simulink model "ChimeIndicatorOutput"  (R2018b)
settings: Solver=FixedStepDiscrete  StartTime=0.0  StopTime=10.0  FixedStep=0.01  RelTol=1e-3
undefined symbols (not defined in the file or in its folder): f, h, IfVeSMSeStNumConfig, KeSMSbMdChime1Enable_Val, KeSMSbSRSPosNumConfig_Val, KeSMSuChmReqDurmTm_Val, KeSMSuChmReqIntlTm_Val, KeSMSwModeChimeReqTm_Val, KeSMSwSRSActiveValidTm_Val, SRSIndicatorStat1
libraries: MSMLib x27
(part 2 of 2)

== stateflow chart ChimeIndicatorOutput/ChimeIndicatorOutputRunnable_sys/Subsystem/SRSIndicator/Chart ==
  state PowerOn
  state Slct_None
    en:
    oSRSIndicatorStat = SRSIndicatorStat1.SRSIndicatorStat1_NoIndicator;
    oSRSMdSlctSwStat =0;
    oSRSMdSlctSwIndTyp = 0;
  state Slct_Avail
    state NotConfirm
      state ON
        en:
        oSRSIndicatorStat = iSlctSwStat;
        oSRSMdSlctSwStat = iSRSMdSlctSwReq_67_2;
        oSRSMdSlctSwIndTyp = 3;
      state OFF
        en:
        oSRSIndicatorStat = SRSIndicatorStat1.SRSIndicatorStat1_NoIndicator;
        oSRSMdSlctSwStat = 0;
        oSRSMdSlctSwIndTyp = 0;
      Slct_Avail.NotConfirm.ON -> Slct_Avail.NotConfirm.ON [order 2] : [hasChanged(iSlctSwStat) && (iSlctSwStat != SRSIndicatorStat1.SRSIndicatorStat1_NoIndicator)]
      Slct_Avail.NotConfirm.ON -> Slct_Avail.NotConfirm.OFF [order 3] : [after(iValideTm,tick)]
      (default) -> Slct_Avail.NotConfirm.ON
      Slct_Avail.NotConfirm.OFF -> Slct_Avail.NotConfirm.ON : [hasChanged(iSlctSwStat)]
    state Confirm
      en:
      oSRSMdSlctSwIndTyp = 1;
      du:
      oSRSIndicatorStat =ConfirmSRSIndicatorStat();
      state ON
        en:
        SRSMdSlctSwReq_67_2_temp = iSRSMdSlctSwReq_67_2;
      state OFF
        en:
        SRSMdSlctSwReq_67_2_temp = 0;
      Slct_Avail.Confirm.ON -> Slct_Avail.Confirm.ON [order 2] : [(iSRSMdSlctSwReq_67_2 != SRSMdSlctSwReq_67_2_temp) && (iSRSMdSlctSwReq_67_2 != 0)]
      (default) -> Slct_Avail.Confirm.OFF
      Slct_Avail.Confirm.OFF -> Slct_Avail.Confirm.ON : [iSRSMdSlctSwReq_67_2 != 0]
      Slct_Avail.Confirm.ON -> Slct_Avail.Confirm.OFF [order 1] : [after(iValideTm,tick)]
    (default) -> NotConfirm
    Confirm -> Slct_Avail.NotConfirm.OFF [order 2] : [(icurMode == MdTp1.MdTp_None)&&after(5,tick)]
    Slct_Avail.NotConfirm.ON -> Confirm [order 1] : [hasChangedTo(iIsActive,true)]
  note: // fail to start Mode for Avl invalid
  state out =ConfirmSRSIndicatorStat [function]
    (default) -> (junction 263)
    (junction 263) -> (junction 264) [order 1] : [iSRSMode == SRSCurMode1.SRSMode_EZEEntry]
    (junction 264) -> (junction 287) : {out = SRSIndicatorStat1.SRSIndicatorStat1_EzeEntry;}
    (junction 263) -> (junction 265) [order 2]
    (junction 265) -> (junction 266) [order 1] : [iSRSMode == SRSCurMode1.SRSMode_EzeExt]
    (junction 266) -> (junction 286) : {out = SRSIndicatorStat1.SRSIndicatorStat1_EzeExit;}
    (junction 265) -> (junction 267) [order 2]
    (junction 267) -> (junction 268) [order 1] : [iSRSMode == SRSCurMode1.SRSMode_LfVip]
    (junction 268) -> (junction 285) : {out = SRSIndicatorStat1.SRSIndicatorStat1_LfVip;}
    (junction 267) -> (junction 269) [order 2]
    (junction 269) -> (junction 270) [order 1] : [iSRSMode == SRSCurMode1.SRSMode_RtVip]
    (junction 270) -> (junction 284) : {out = SRSIndicatorStat1.SRSIndicatorStat1_RtVip;}
    (junction 269) -> (junction 271) [order 2]
    (junction 271) -> (junction 272) [order 1] : [iSRSMode == SRSCurMode1.SRSMode_AllVip]
    (junction 272) -> (junction 283) : {out = SRSIndicatorStat1.SRSIndicatorStat1_AllVip;}
    (junction 271) -> (junction 273) [order 2]
    (junction 273) -> (junction 274) [order 1] : [iSRSMode == SRSCurMode1.SRSMode_LfLug]
    (junction 274) -> (junction 282) : {out = SRSIndicatorStat1.SRSIndicatorStat1_LfLug;}
    (junction 273) -> (junction 275) [order 2]
    (junction 275) -> (junction 276) [order 1] : [iSRSMode == SRSCurMode1.SRSMode_RtLug]
    (junction 276) -> (junction 281) : {out = SRSIndicatorStat1.SRSIndicatorStat1_RtLug;}
    (junction 275) -> (junction 277) [order 2]
    (junction 277) -> (junction 278) [order 1] : [iSRSMode == SRSCurMode1.SRSMode_AllLug]
    (junction 278) -> (junction 280) : {out = SRSIndicatorStat1.SRSIndicatorStat1_AllLug;}
    (junction 277) -> (junction 387) [order 2]
    (junction 387) -> (junction 386) [order 1] : [iSRSMode == SRSCurMode1.SRSMode_IntimacyL]
    (junction 386) -> (junction 390) : {out = SRSIndicatorStat1.SRSIndicatorStat1_IntimacyL;}
    (junction 387) -> (junction 393) [order 2]
    (junction 393) -> (junction 395) [order 1] : [iSRSMode == SRSCurMode1.SRSMode_FamilyR]
    (junction 395) -> (junction 397) : {out = SRSIndicatorStat1.SRSIndicatorStat1_FamilyR;}
    (junction 393) -> (junction 400) [order 2]
    (junction 400) -> (junction 402) [order 1] : [iSRSMode == SRSCurMode1.SRSMode_FamilyL]
    (junction 402) -> (junction 404) : {out = SRSIndicatorStat1.SRSIndicatorStat1_FamilyL;}
    (junction 400) -> (junction 407) [order 2]
    (junction 407) -> (junction 409) [order 1] : [iSRSMode == SRSCurMode1.SRSMode_RcvyL]
    (junction 409) -> (junction 411) : {out = SRSIndicatorStat1.SRSIndicatorStat1_RcvyL;}
    (junction 407) -> (junction 414) [order 2]
    (junction 414) -> (junction 416) [order 1] : [iSRSMode == SRSCurMode1.SRSMode_RcvyR]
    (junction 416) -> (junction 418) : {out = SRSIndicatorStat1.SRSIndicatorStat1_RcvyR;}
    (junction 414) -> (junction 421) [order 2]
    (junction 421) -> (junction 423) [order 1] : [iSRSMode == SRSCurMode1.SRSMode_LyingL]
    (junction 423) -> (junction 425) : {out = SRSIndicatorStat1.SRSIndicatorStat1_LyingL;}
    (junction 421) -> (junction 430) [order 2]
    (junction 430) -> (junction 429) [order 1] : [iSRSMode == SRSCurMode1.SRSMode_LyingR]
    (junction 429) -> (junction 433) : {out = SRSIndicatorStat1.SRSIndicatorStat1_LyingR;}
    (junction 430) -> (junction 437) [order 2]
    (junction 437) -> (junction 439) [order 1] : [iSRSMode == SRSCurMode1.SRSMode_LgrstOpenLt]
    (junction 439) -> (junction 441) : {out = SRSIndicatorStat1.SRSIndicatorStat1_LgrstOpenLt;}
    (junction 437) -> (junction 444) [order 2]
    (junction 444) -> (junction 446) [order 1] : [iSRSMode == SRSCurMode1.SRSMode_LgrstCloseLt]
    (junction 446) -> (junction 448) : {out = SRSIndicatorStat1.SRSIndicatorStat1_LgrstCloseLt;}
    (junction 444) -> (junction 451) [order 2]
    (junction 451) -> (junction 453) [order 1] : [iSRSMode == SRSCurMode1.SRSMode_LgrstOpenRt]
    (junction 453) -> (junction 455) : {out = SRSIndicatorStat1.SRSIndicatorStat1_LgrstOpenRt;}
    (junction 451) -> (junction 458) [order 2]
    (junction 458) -> (junction 460) [order 1] : [iSRSMode == SRSCurMode1.SRSMode_LgrstCloseRt]
    (junction 460) -> (junction 462) : {out = SRSIndicatorStat1.SRSIndicatorStat1_LgrstCloseRt;}
    (junction 458) -> (junction 465) [order 2]
    (junction 465) -> (junction 467) [order 1] : [iSRSMode == SRSCurMode1.SRSMode_IntimacyR]
    (junction 467) -> (junction 468) : {out = SRSIndicatorStat1.SRSIndicatorStat1_IntimacyR;}
    (junction 465) -> (junction 543) [order 2]
    (junction 543) -> (junction 545) [order 1] : [iSRSMode == SRSCurMode1.SRSMode_EzeEntry4s2L]
    (junction 545) -> (junction 548) : {out = SRSIndicatorStat1.SRSIndicatorStat1_EzeEntry4s2L;}
    (junction 543) -> (junction 551) [order 2]
    (junction 551) -> (junction 553) [order 1] : [iSRSMode == SRSCurMode1.SRSMode_EzeExt4s2L]
    (junction 553) -> (junction 555) : {out = SRSIndicatorStat1.SRSIndicatorStat1_EzeExt4s2L;}
    (junction 551) -> (junction 558) [order 2]
    (junction 558) -> (junction 560) [order 1] : [iSRSMode == SRSCurMode1.SRSMode_EzeEntry4s2R]
    (junction 558) -> (junction 565) [order 2]
    (junction 560) -> (junction 562) : {out = SRSIndicatorStat1.SRSIndicatorStat1_EzeEntry4s2R;}
    (junction 565) -> (junction 567) [order 1] : [iSRSMode == SRSCurMode1.SRSMode_EzeExt4s2R]
    (junction 565) -> (junction 572) [order 2]
    (junction 567) -> (junction 569) : {out = SRSIndicatorStat1.SRSIndicatorStat1_EzeExt4s2R;}
    (junction 572) -> (junction 574) [order 1] : [iSRSMode == SRSCurMode1.SRSMode_EzeEntryAll4sBwd]
    (junction 572) -> (junction 579) [order 2]
    (junction 574) -> (junction 576) : {out = SRSIndicatorStat1.SRSIndicatorStat1_EzeEntryAll4sBwd;}
    (junction 579) -> (junction 581) [order 1] : [iSRSMode == SRSCurMode1.SRSMode_EzeEntryAll4sFwd]
    (junction 579) -> (junction 279) [order 2] : {out = SRSIndicatorStat1.SRSIndicatorStat1_NoIndicator;}
    (junction 581) -> (junction 583) : {out = SRSIndicatorStat1.SRSIndicatorStat1_EzeEntryAll4sFwd;}
    (junction 462) -> (junction 468)
    (junction 455) -> (junction 462)
    (junction 448) -> (junction 455)
    (junction 441) -> (junction 448)
    (junction 433) -> (junction 441)
    (junction 425) -> (junction 433)
    (junction 418) -> (junction 425)
    (junction 411) -> (junction 418)
    (junction 404) -> (junction 411)
    (junction 397) -> (junction 404)
    (junction 390) -> (junction 397)
    (junction 280) -> (junction 390)
    (junction 281) -> (junction 280)
    (junction 282) -> (junction 281)
    (junction 283) -> (junction 282)
    (junction 284) -> (junction 283)
    (junction 285) -> (junction 284)
    (junction 286) -> (junction 285)
    (junction 287) -> (junction 286)
    (junction 468) -> (junction 548)
    (junction 548) -> (junction 555)
    (junction 555) -> (junction 562)
    (junction 583) -> (junction 279)
    (junction 576) -> (junction 583)
    (junction 569) -> (junction 576)
    (junction 562) -> (junction 569)
    (junction 279) -> (junction 288)
  note: //mode ending or Interrupt
  (default) -> PowerOn
  PowerOn -> Slct_None : [after(10,tick)]
  Slct_None -> NotConfirm [order 1] : [hasChangedFrom(iSlctSwStat,SRSIndicatorStat1.SRSIndicatorStat1_NoIndicator)]
  Slct_None -> Confirm [order 2] : [(SRSMdSlctSwReq_67_2_temp != 0) && hasChangedTo(iIsActive,true)]
      | {oSRSMdSlctSwStat = SRSMdSlctSwReq_67_2_temp;}
  Confirm -> Slct_None [order 1] : [hasChangedTo(icurMode, MdTp1.MdTp_None)]
  data: out function_output Enum: SRSIndicatorStat1; iSlctSwStat input Enum: SRSIndicatorStat1; oSRSIndicatorStat output Enum: SRSIndicatorStat1; iIsActive input boolean; iValideTm input uint16; iSlctSwStat_last local Enum: SRSIndicatorStat1; icurMode input; iSRSMode input Enum: SRSCurMode1; iSRSMdSlctSwReq_67_2 input uint8; oSRSMdSlctSwStat output uint8; oSRSMdSlctSwIndTyp output Enum: SRSSlctSwIndTyp; SRSMdSlctSwReq_67_2_temp local uint8
